simulink model "stateflow_example"  (Simulink 8.0)
settings: Solver=FixedStepDiscrete  StartTime=0.0  StopTime=10.0  RelTol=1e-3
settings Model: Creator=rstarr  LastModifiedBy=rstarr

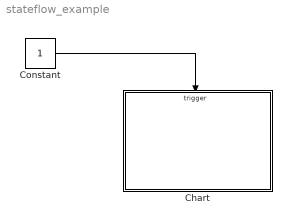
== system stateflow_example ==
  Chart : Stateflow chart  TreatAsAtomicUnit=on
  Constant : Constant
  wires:
  Constant/1 -> Chart/Trigger

== stateflow chart Chart ==
  state Initial
  state Final
  Initial -> Final : event
  (default) -> Initial
  events: event input RISING_EDGE_EVENT
